simulink model "carsim_template_v1"  (R2022b)
settings: Solver=ode4  StartTime=0.0  StopTime=10  FixedStep=0.01  RelTol=1e-3
settings Model: Creator=ranwe  LastModifiedBy=ranwe

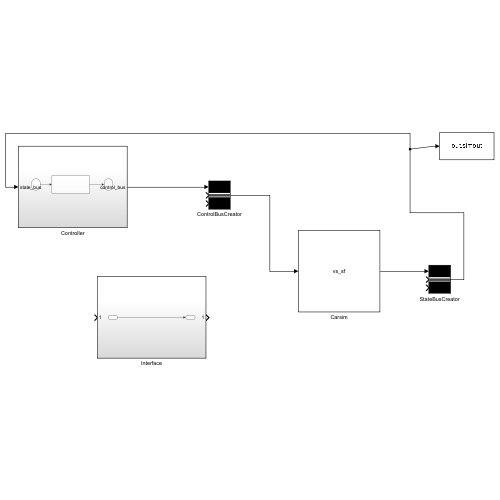
[thumbnail: Simulink's stored preview of the top-level diagram]
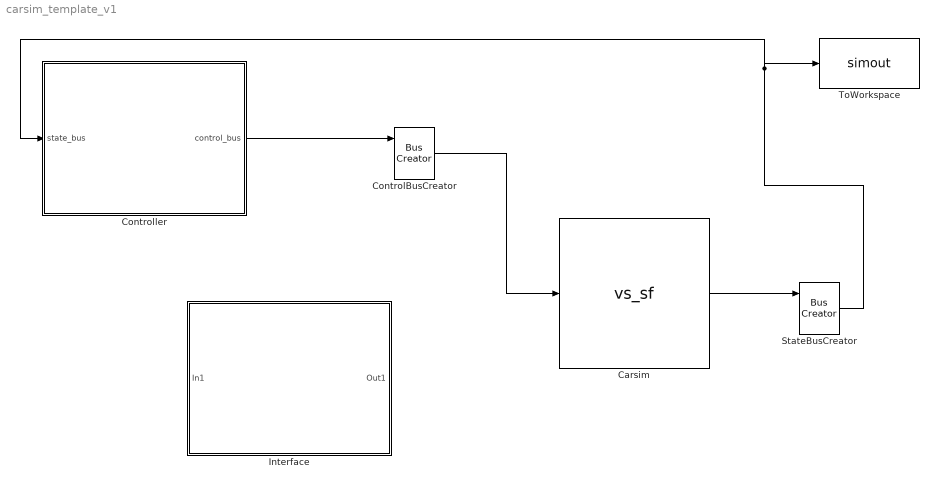
== system carsim_template_v1 ==
  Carsim : S-Function  FunctionName=vs_sf  Parameters=simfile.sim  SFunctionDeploymentMode=off  EnableBusSupport=off
  ControlBusCreator : BusCreator  Inputs=3
  Controller : Subsystem
  Interface : Subsystem
  StateBusCreator : BusCreator  Inputs=3
  ToWorkspace : ToWorkspace  VariableName=simout  SaveFormat=Structure With Time  SampleTime=-1
  wires:
  Controller/1(control_bus) -> ControlBusCreator/1
  ControlBusCreator/1 -> Carsim/1
  Carsim/1 -> StateBusCreator/1
  StateBusCreator/1 -> ToWorkspace/1, Controller/1(state_bus)

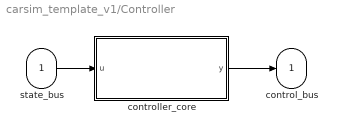
== system carsim_template_v1/Controller ==
  state_bus : Inport
  controller_core : MATLAB Function  TreatAsAtomicUnit=on
  control_bus : Outport
  wires:
  state_bus/1 -> controller_core/1(u)
  controller_core/1(y) -> control_bus/1

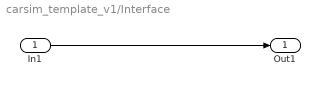
== system carsim_template_v1/Interface ==
  In1 : Inport
  Out1 : Outport
  wires:
  In1/1 -> Out1/1

== matlab function carsim_template_v1/Controller/controller_core ==
  data: u input; y output
function y = fcn(u)

y = u;
